simulink model "FF_Controller"  (R2022b)
settings: Solver=FixedStepAuto  StartTime=0.0  StopTime=10.0  FixedStep=.005  RelTol=1e-3
undefined symbols (not defined in the file or in its folder): angular, linear
libraries: ros2lib x9
settings Model: Creator=hollis  LastModifiedBy=hollis
settings OptimizationCC: EnhancedBackFolding=on  PassReuseOutputArgsAs=Individual arguments  ZeroExternalMemoryAtStartup=off  ZeroInternalMemoryAtStartup=off  MaxStackSize=64  OptimizeBlockOrder=speed  DifferentSizesBufferReuse=on  OptimizationCustomize=off  EfficientTunableParamExpr=on
settings DebuggingCC: ParameterTunabilityLossMsg=error
settings HardwareCC: ProdLargestAtomicInteger=Long  ProdLargestAtomicFloat=Double  ProdLongLongMode=on  ProdHWDeviceType=ARM Compatible->ARM 64-bit (LLP64)
settings SFSimCC: MATLABDynamicMemAlloc=off
settings RTWCC: Description=Embedded Coder  SystemTargetFile=ert.tlc  HardwareBoard=Robot Operating System 2 (ROS 2)  TLCOptions="-aInlineSetEventsForThisBaseRateFcn=TLC_FALSE -aSuppressMultiTaskScheduler=TLC_FALSE  -aRateBasedStepFcn=0"  TemplateMakefile=ert_default_tmf  Toolchain=Colcon Tools  BuildConfiguration=Faster Runs  TargetLang=C++
settings CodeAppCC: ForceParamTrailComments=on  IgnoreCustomStorageClasses=off  OperatorAnnotations=on  SimulinkDataObjDesc=on  SFDataObjDesc=on  InsertBlockDesc=on
settings ERTTargetCC: CodeInterfacePackaging=C++ class  SupportVariableSizeSignals=on  RootIOFormat=Structure reference

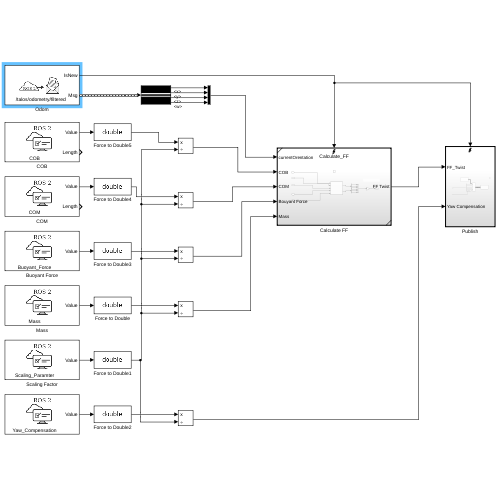
[thumbnail: Simulink's stored preview of the top-level diagram]
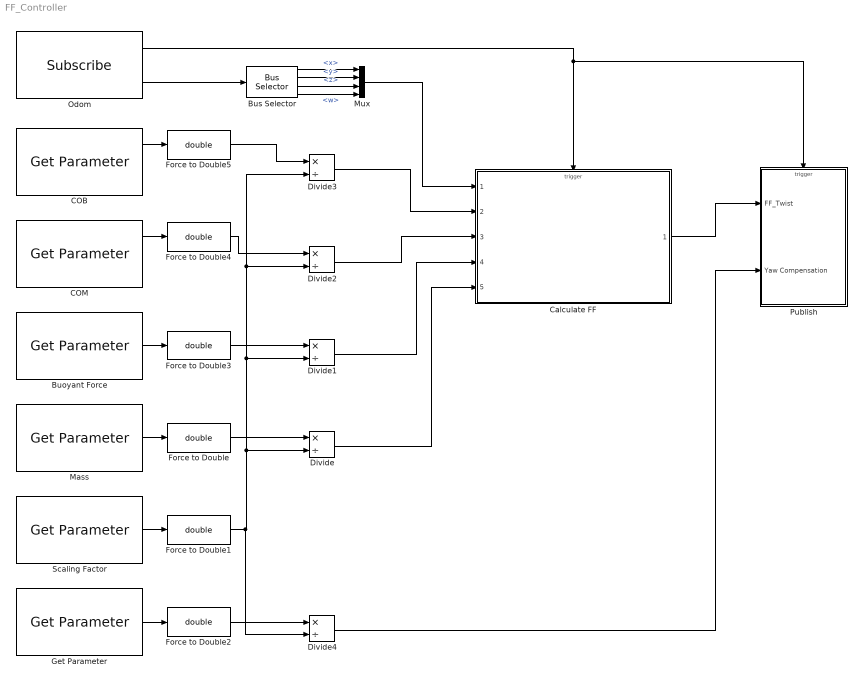
== system FF_Controller ==
  Buoyant Force : ros2lib/Get Parameter  ParameterName=Buoyant_Force  ParameterType=int64  ParameterMaxArrayLength=16  ParameterInitialValue=0.0  SampleTime=-1  ModelName=FF_Controller  BlockId=ParamGet_FF_Controller_69
      settings: LibrarySourceBlock=roslib/ROS 2/Get Parameter
  Bus Selector : BusSelector  OutputSignals=pose.pose.orientation.x,pose.pose.orientation.y,pose.pose.orientation.z,pose.pose.orientation.w
  COB : ros2lib/Get Parameter  ParameterName=COB  ParameterType=int64[]  ParameterMaxArrayLength=3  ParameterInitialValue=[0,0,0]  SampleTime=-1  ModelName=FF_Controller  BlockId=ParamGet_FF_Controller_67
      settings: LibrarySourceBlock=roslib/ROS 2/Get Parameter
  COM : ros2lib/Get Parameter  ParameterName=COM  ParameterType=int64[]  ParameterMaxArrayLength=3  ParameterInitialValue=[0,0,0]  SampleTime=-1  ModelName=FF_Controller  BlockId=ParamGet_FF_Controller_68
      settings: LibrarySourceBlock=roslib/ROS 2/Get Parameter
  Calculate FF : Subsystem  ReferencedSubsystem=Calculate_FF
  Divide{,1..4} (5 alike) : Product  Inputs=*/
  Force to Double{,1..5} (6 alike) : DataTypeConversion  OutDataTypeStr=double  SaturateOnIntegerOverflow=off  RndMeth=Floor
  Get Parameter : ros2lib/Get Parameter  ParameterName=Yaw_Compensation  ParameterType=int64  ParameterMaxArrayLength=16  ParameterInitialValue=0.0  SampleTime=-1  ModelName=FF_Controller  BlockId=ParamGet_FF_Controller_80
      settings: LibrarySourceBlock=roslib/ROS 2/Get Parameter
  Mass : ros2lib/Get Parameter  ParameterName=Mass  ParameterType=int64  ParameterMaxArrayLength=16  ParameterInitialValue=0.0  SampleTime=-1  ModelName=FF_Controller  BlockId=ParamGet_FF_Controller_70
      settings: LibrarySourceBlock=roslib/ROS 2/Get Parameter
  Mux : Mux
  Odom : ros2lib/Subscribe  topicSource=Specify your own  topic=/talos/odometry/filtered  messageType=nav_msgs/Odometry  sampleTime=-1  QOSHistory=Keep last  QOSDepth=1  QOSReliability=Reliable  QOSDurability=Volatile
      settings: LibrarySourceBlock=roslib/ROS 2/Subscribe
  Publish : Subsystem
  Scaling Factor : ros2lib/Get Parameter  ParameterName=Scaling_Paramter  ParameterType=int64  ParameterMaxArrayLength=16  ParameterInitialValue=1  SampleTime=-1  ModelName=FF_Controller  BlockId=ParamGet_FF_Controller_71
      settings: LibrarySourceBlock=roslib/ROS 2/Get Parameter
  wires:
  Calculate FF/1 -> Publish/1(FF_Twist)
  Odom/2 -> Bus Selector/1
  Odom/1 -> Publish/Trigger, Calculate FF/Trigger
  Bus Selector/1 -> Mux/1  "<x>"
  Bus Selector/2 -> Mux/2  "<y>"
  Bus Selector/3 -> Mux/3  "<z>"
  Bus Selector/4 -> Mux/4  "<w>"
  Mux/1 -> Calculate FF/1
  Buoyant Force/1 -> Force to Double3/1
  Mass/1 -> Force to Double/1
  Divide3/1 -> Calculate FF/2
  Divide2/1 -> Calculate FF/3
  Divide1/1 -> Calculate FF/4
  Divide/1 -> Calculate FF/5
  Scaling Factor/1 -> Force to Double1/1
  Get Parameter/1 -> Force to Double2/1
  Divide4/1 -> Publish/2(Yaw Compensation)
  Force to Double/1 -> Divide/1
  Force to Double1/1 -> Divide3/2, Divide2/2, Divide1/2, Divide/2, Divide4/2
  Force to Double2/1 -> Divide4/1
  Force to Double3/1 -> Divide1/1
  COM/1 -> Force to Double4/1
  Force to Double4/1 -> Divide2/1
  COB/1 -> Force to Double5/1
  Force to Double5/1 -> Divide3/1

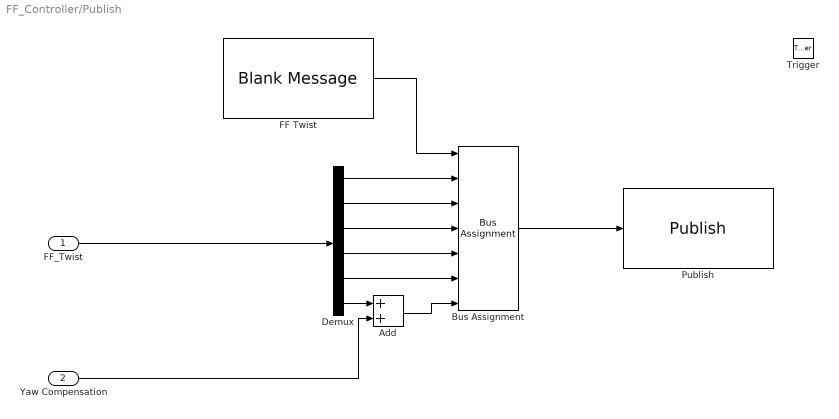
== system FF_Controller/Publish ==
  FF_Twist : Inport
  Yaw Compensation : Inport  Port=2
  Trigger : TriggerPort  VariantControl=(inherit)  PortDimensions=1
  Add : Sum
  Bus Assignment : BusAssignment  AssignedSignals=linear.x,linear.y,linear.z,angular.x,angular.y,angular.z
  Demux : Demux  Outputs=6
  FF Twist : ros2lib/Blank Message  messageClass=Message  entityType=geometry_msgs/Twist  messageType=geometry_msgs/Twist  SampleTime=inf
      settings: LibrarySourceBlock=roslib/ROS 2/Blank Message
  Publish : ros2lib/Publish  topicSource=Specify your own  topic=/talos/controller/FF_body_force  messageType=geometry_msgs/Twist  QOSHistory=Keep last  QOSDepth=1  QOSReliability=Reliable  QOSDurability=Volatile
      settings: LibrarySourceBlock=roslib/ROS 2/Publish
  wires:
  Bus Assignment/1 -> Publish/1
  FF Twist/1 -> Bus Assignment/1
  Demux/1 -> Bus Assignment/2
  Demux/2 -> Bus Assignment/3
  Demux/3 -> Bus Assignment/4
  Demux/4 -> Bus Assignment/5
  Demux/5 -> Bus Assignment/6
  FF_Twist/1 -> Demux/1
  Yaw Compensation/1 -> Add/2
  Demux/6 -> Add/1
  Add/1 -> Bus Assignment/7
